simulink library "uram_lib"  (R2013b)
settings: Solver=ode45  SolverMode=SingleTasking  StartTime=0.0  StopTime=10.0  RelTol=1e-3
libraries: xbsIndex_r4 x4
settings Model: CovMetricSettings=dwe  CovHtmlReporting=off  covSaveCumulativeToWorkspaceVar=off  CovSaveSingleToWorkspaceVar=off  CovExternalEMLEnable=on  Creator=Administrator  LastModifiedBy=Administrator

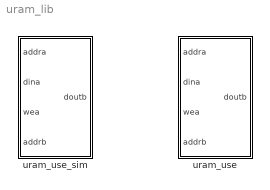
== system uram_lib ==
  uram_use : Subsystem
  uram_use_sim : Subsystem

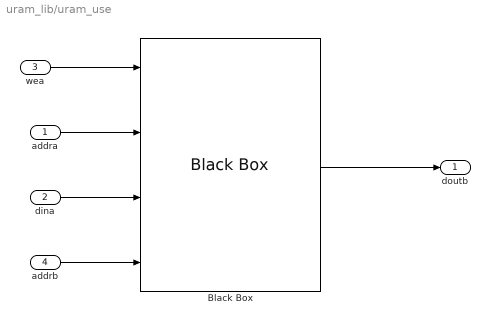
== system uram_lib/uram_use ==
  addra : Inport
  dina : Inport  Port=2
  wea : Inport  Port=3
  addrb : Inport  Port=4
  Black Box : xbsIndex_r4/Black Box  init_code=uram32k_wrapper_config  sim_method=ISE Simulator  verbose=off  block_type=blackbox2
  doutb : Outport
  wires:
  addrb/1 -> Black Box/4
  Black Box/1 -> doutb/1
  wea/1 -> Black Box/1
  dina/1 -> Black Box/3
  addra/1 -> Black Box/2

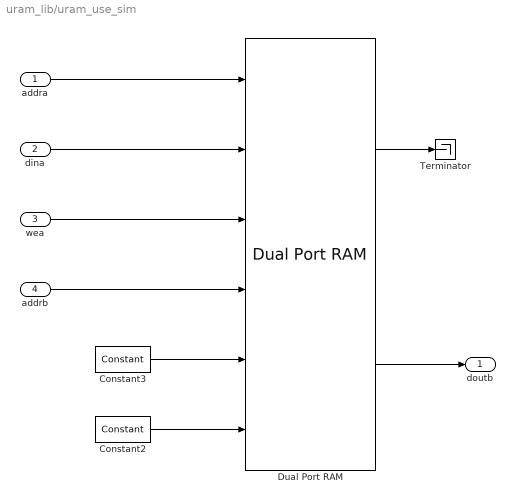
== system uram_lib/uram_use_sim ==
  addra : Inport
  dina : Inport  Port=2
  wea : Inport  Port=3
  addrb : Inport  Port=4
  Constant2 : xbsIndex_r4/Constant  const=0  gui_display_data_type=Boolean  arith_type=Boolean  n_bits=2  bin_pt=0  preci_type=Single  exp_width=8  frac_width=24  explicit_period=off  period=1  equ=P=C  opselect=C  inp2=PCIN>>17  opr=+  inp1=P  carry=CIN  dbl_ovrd=off  block_type=constant
  Constant3 : xbsIndex_r4/Constant  const=0  gui_display_data_type=Fixed-point  arith_type=Unsigned  n_bits=64  bin_pt=0  preci_type=Single  exp_width=8  frac_width=24  explicit_period=off  period=1  equ=P=C  opselect=C  inp2=PCIN>>17  opr=+  inp1=P  carry=CIN  dbl_ovrd=off  block_type=constant
  Dual Port RAM : xbsIndex_r4/Dual Port RAM  depth=32768  initVector=0  distributed_mem=Ultra RAM  init_a=0  init_b=0  rst_a=off  rst_b=off  en_a=off  en_b=off  latency=10  write_mode_A=Read After Write  write_mode_B=Read After Write  optimize=Area  dbl_ovrd=off  block_type=dpram
  Terminator : Terminator
  doutb : Outport
  wires:
  addrb/1 -> Dual Port RAM/4
  wea/1 -> Dual Port RAM/3
  dina/1 -> Dual Port RAM/2
  addra/1 -> Dual Port RAM/1
  Constant2/1 -> Dual Port RAM/6
  Dual Port RAM/2 -> doutb/1
  Dual Port RAM/1 -> Terminator/1
  Constant3/1 -> Dual Port RAM/5
